simulink model "konstelacja"  (R2016a)
settings: Solver=FixedStepDiscrete  StartTime=0.0  StopTime=inf  RelTol=1e-3
libraries: commfilt2 x2, commdigbbndpm3 x1, dspsigops x1, commrandsrc2 x1, commutil2 x1
settings Model: Creator=sikor  LastModifiedBy=sikor
settings DataIOCC: LimitDataPoints=on  SaveFormat=Array
settings DebuggingCC: SolverPrmCheckMsg=warning
settings HardwareCC: ProdBitPerPointer=32  ProdLargestAtomicFloat=None  ProdIntDivRoundTo=Undefined  ProdEndianess=Unspecified  ProdWordSize=32  ProdHWDeviceType=32-bit Generic
settings ModelReferenceCC: PropagateSignalLabelsOutOfModel=off
settings ConfigComp: CovModelRefEnable=Off  CovSFcnEnable=off

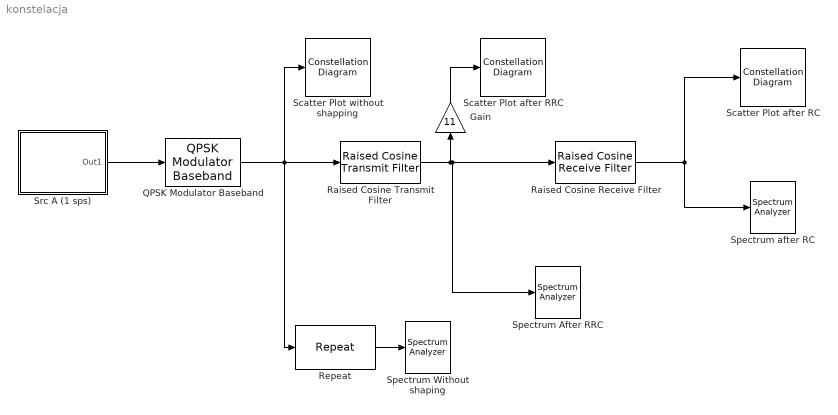
== system konstelacja ==
  Gain : Gain  Gain=11
  QPSK Modulator Baseband : commdigbbndpm3/QPSK Modulator Baseband  InType=Integer  Enc=Gray  Ph=pi/4  outDtype=double  outWordLen=16  outUDDataType=sfix(16)  outFracLenMode=Best precision  outFracLen=15  outDataTypeStr=double  outLastDataTypeStr=double
  Raised Cosine Receive Filter : commfilt2/Raised Cosine Receive Filter  filtType=Square root  R=0.2  filtSpan=10  N=128  downFactor=1  downOffset=0  filterGain=1  InputProcessing=Columns as channels (frame based)  RateOptions=Allow multirate processing  framing=Mute  checkCoeff=off  variableName=rcRxFilt  currentFiltSpan=10  D=5  inputOffset=0  sampMode=Mute  saveAsFlag=0  rateMode=Downsampling  checkGain=Normalized  launchFVT=on  roundingMode=Floor  overflowMode=off  coeffDataTypeStr=Inherit: Same word length as input  coeffMin=[]  coeffMax=[]  coeffLastDataTypeStr=Inherit: Same word length as input  accumDataTypeStr=Inherit: Same as product output  accumLastDataTypeStr=Inherit: Same as product output  outputDataTypeStr=Inherit: Same as accumulator  outputMin=[]  outputMax=[]  outputLastDataTypeStr=Inherit: Same as accumulator
  Raised Cosine Transmit Filter : commfilt2/Raised Cosine Transmit Filter  filtType=Square root  R=0.2  filtSpan=10  N=128  filterGain=1  InputProcessing=Columns as channels (frame based)  RateOptions=Allow multirate processing  framing=Mute  checkCoeff=off  variableName=rcTxFilt  checkGain=Normalized  sampMode=Mute  saveAsFlag=0  currentFiltSpan=10  D=(10)/2  launchFVT=on  roundingMode=Floor  overflowMode=off  coeffDataTypeStr=Inherit: Same word length as input  coeffMin=[]  coeffMax=[]  coeffLastDataTypeStr=Inherit: Same word length as input  outputDataTypeStr=Inherit: Same as accumulator  outputMin=[]  outputMax=[]  outputLastDataTypeStr=Inherit: Same as accumulator
  Repeat : dspsigops/Repeat  N=100  InputProcessing=Columns as channels (frame based)  RateOptions=Allow multirate processing  ic=0  mode=Unused parameter value
  Scatter Plot after RC : ConstellationDiagram  Tag=ScatterPlot
  Scatter Plot after RRC : ConstellationDiagram  Tag=ScatterPlot
  Scatter Plot without shapping : ConstellationDiagram  Tag=ScatterPlot
  Spectrum After RRC : SpectrumAnalyzer
  Spectrum Without shaping : SpectrumAnalyzer
  Spectrum after RC : SpectrumAnalyzer
  Src A (1 sps) : Subsystem
  wires:
  Src A (1 sps)/1(Out1) -> QPSK Modulator Baseband/1
  QPSK Modulator Baseband/1 -> Repeat/1, Scatter Plot without shapping/1, Raised Cosine Transmit Filter/1
  Raised Cosine Receive Filter/1 -> Scatter Plot after RC/1, Spectrum after RC/1
  Raised Cosine Transmit Filter/1 -> Spectrum After RRC/1, Raised Cosine Receive Filter/1, Gain/1
  Gain/1 -> Scatter Plot after RRC/1
  Repeat/1 -> Spectrum Without shaping/1

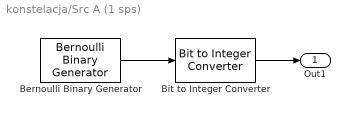
== system konstelacja/Src A (1 sps) ==
  Bernoulli Binary Generator : commrandsrc2/Bernoulli Binary Generator  P=0.5  seed=61  Ts=0.5  frameBased=on  sampPerFrame=2  orient=off  outDataType=boolean
  Bit to Integer Converter : commutil2/Bit to Integer Converter  nbits=2  bitOrder=MSB first  signedOutputValues=Unsigned  outDtype=int16  outDtypeSigned=Inherit via internal rule
  Out1 : Outport
  wires:
  Bernoulli Binary Generator/1 -> Bit to Integer Converter/1
  Bit to Integer Converter/1 -> Out1/1
